simulink model "Boeing787_OldMission_ElectricalThermalHydraulicFuelECS"  (R2013a)
settings: Solver=ode23tb  SolverMode=SingleTasking  StartTime=0.0  StopTime=346  RelTol=1e-3
InitFcn:
  | load('SampleOutput.mat')
  | 
  | load('SampleFuelBurn.mat')
undefined symbols (not defined in the file or in its folder): ailerons, AirProp, B_737, elevator, FuelBurn, HydProp, landing_gear, rudder, thrust_rev
libraries: PowerFlowLib x118, simulink x20
(part 26 of 26)

== system Boeing787_OldMission_ElectricalThermalHydraulicFuelECS/ECS/Left Pack/Secondary HX (air-air)1/Air_properties_in_flows_hot_and_cold/air_properties_in_hot ==
  note: PLEASE NOTE that the air properties are based on the
      | inlet flow conditions rather than the average T and P.
      | Trying to base the properties on the average temperature
      | and even a constant pressure, the program did not work. One
      | suggestion is to average the inlet conditions with the outlet conditions
      | at a previous time step by using a memory block.x
  In_flow_bus_hot : Inport
  Bus Selector : BusSelector  OutputSignals=pres_Pa,temp_C
  C to K : Bias  Bias=273
  Cp(P,T) : Lookup_n-D  BreakpointsForDimension1=AirProp.P  BreakpointsForDimension2=AirProp.T  BreakpointsForDimension3=[1]  Table=AirProp.Cp_pt  RndMeth=Simplest  InputSameDT=on
  Cp_pt_hot : Display
  Gain : Gain  Gain=1000
  Pa to kPa : Gain  Gain=10^-3
  Pr(P,T) : Lookup_n-D  BreakpointsForDimension1=AirProp.P  BreakpointsForDimension2=AirProp.T  BreakpointsForDimension3=[1]  Table=AirProp.Pr_pt  RndMeth=Simplest  InputSameDT=on
  Pr_pt_hot : Display
  Rho(P,T) : Lookup_n-D  BreakpointsForDimension1=AirProp.P  BreakpointsForDimension2=AirProp.T  BreakpointsForDimension3=[1]  Table=AirProp.Rho_pt  RndMeth=Simplest  InputSameDT=on
  Rho_pt_hot : Display
  k(P,T) : Lookup_n-D  BreakpointsForDimension1=AirProp.P  BreakpointsForDimension2=AirProp.T  BreakpointsForDimension3=[1]  Table=AirProp.k_pt  RndMeth=Simplest  InputSameDT=on
  k_pt_hot : Display
  mu(P,T) : Lookup_n-D  BreakpointsForDimension1=AirProp.P  BreakpointsForDimension2=AirProp.T  BreakpointsForDimension3=[1]  Table=AirProp.mu_pt  RndMeth=Simplest  InputSameDT=on
  mu_pt_hot : Display
  rho_air_kgm-3 : Outport
  cp_air_Jkg-1K-1 : Outport  Port=2
  mu_air_Pa.s : Outport  Port=3
  K_air_Wm-1K-2 : Outport  Port=4
  Pr : Outport  Port=5
  wires:
  In_flow_bus_hot/1 -> Bus Selector/1
  C to K/1 -> Rho(P,T)/2, Pr(P,T)/2, k(P,T)/2, mu(P,T)/2, Cp(P,T)/2
  Bus Selector/1 -> Pa to kPa/1  "<pres_Pa>"
  Bus Selector/2 -> C to K/1  "<temp_C>"
  Pa to kPa/1 -> Rho(P,T)/1, Cp(P,T)/1, mu(P,T)/1, Pr(P,T)/1, k(P,T)/1  "press_kPa"
  Rho(P,T)/1 -> Rho_pt_hot/1, rho_air_kgm-3/1
  Pr(P,T)/1 -> Pr/1, Pr_pt_hot/1
  k(P,T)/1 -> K_air_Wm-1K-2/1, k_pt_hot/1
  mu(P,T)/1 -> mu_air_Pa.s/1, mu_pt_hot/1
  Cp(P,T)/1 -> Gain/1, Cp_pt_hot/1
  Gain/1 -> cp_air_Jkg-1K-1/1

== system Boeing787_OldMission_ElectricalThermalHydraulicFuelECS/ECS/Left Pack/Secondary HX (air-air)1/HX_and_Fin_paramters/Fin_parameters ==
  Constant : Constant  Value=l_fin
  Constant1 : Constant  Value=t_fin
  Constant2 : Constant  Value=s_fin
  Constant3 : Constant  Value=h_fin
  Constant4 : Constant  Value=K_n
  Constant5 : Constant  Value=eta_f
  Fin_length_m : Outport
  Fin_thickness_m : Outport  Port=2
  Fin_free_flow_width_m : Outport  Port=3
  Fin_free_flow_height_m : Outport  Port=4
  K_fin_Wm-1K-1 : Outport  Port=5
  Fin_eff : Outport  Port=6
  wires:
  Constant1/1 -> Fin_thickness_m/1
  Constant2/1 -> Fin_free_flow_width_m/1
  Constant3/1 -> Fin_free_flow_height_m/1
  Constant4/1 -> K_fin_Wm-1K-1/1
  Constant5/1 -> Fin_eff/1
  Constant/1 -> Fin_length_m/1

== system Boeing787_OldMission_ElectricalThermalHydraulicFuelECS/ECS/Left Pack/Secondary HX (air-air)1/HX_and_Fin_paramters/HX_parameters ==
  Other_HX_parameters : Inport
  Fin_parameters : Inport  Port=2
  Bus Selector : BusSelector  OutputSignals=L_hx
  Calculating the no of passages per fluid flow : Subsystem
  Calculating the total number of fins per HX per fluid flow : Subsystem
  Calculating total free flow area per flow : Subsystem
  Constant3 : Constant  Value=K_p
  Constant4 : Constant  Value=cp_hx
  Constant5 : Constant  Value=m_cm
  Display : Display
  Display1 : Display
  Display2 : Display
  tot_free_flow_area_m^2 : Outport
  tot_length_in_direc_of_flow_m : Outport  Port=2
  tot_no_of_fins_per_HX_per_flow : Outport  Port=3
  K_hx_Wm-1K-1 : Outport  Port=4
  cp_hx_Jkg-1K-1 : Outport  Port=5
  m_hx_kg : Outport  Port=6
  wires:
  Bus Selector/1 -> tot_length_in_direc_of_flow_m/1  "<L_hx>"
  Calculating the total number of fins per HX per fluid flow/1(Tot_no_of_fins_per_HX_per_flow) -> Display2/1, tot_no_of_fins_per_HX_per_flow/1  "N_f"
  Calculating total free flow area per flow/1(Total_free_flow_area) -> Display/1, tot_free_flow_area_m^2/1  "A"
  Calculating the no of passages per fluid flow/1(N_passages_per_flow) -> Display1/1, Calculating the total number of fins per HX per fluid flow/3(N_passages_per_flow), Calculating total free flow area per flow/3(N_passages_per_flow)
  Fin_parameters/1 -> Calculating the total number of fins per HX per fluid flow/2(Fin_parameters), Calculating total free flow area per flow/2(Fin_parameters), Calculating the no of passages per fluid flow/2(Fin_parameters)
  Other_HX_parameters/1 -> Bus Selector/1, Calculating the total number of fins per HX per fluid flow/1(Raw_HX_parameters), Calculating total free flow area per flow/1(Raw_HX_parameters), Calculating the no of passages per fluid flow/1(Raw_HX_parameters)
  Constant5/1 -> m_hx_kg/1
  Constant3/1 -> K_hx_Wm-1K-1/1
  Constant4/1 -> cp_hx_Jkg-1K-1/1

== system Boeing787_OldMission_ElectricalThermalHydraulicFuelECS/ECS/Left Pack/Secondary HX (air-air)1/HX_and_Fin_paramters/Other_HX_parameters2 ==
  Bus Creator : BusCreator
  Length in flow direction : Constant  Value=L_hx
  plate thickness : Constant  Value=t_p
  total height : Constant  Value=H_hx
  width : Constant  Value=W_hx
  Out1 : Outport
  wires:
  Bus Creator/1 -> Out1/1
  plate thickness/1 -> Bus Creator/4  "t_p"
  total height/1 -> Bus Creator/3  "H_hx"
  width/1 -> Bus Creator/2  "W_hx"
  Length in flow direction/1 -> Bus Creator/1  "L_hx"

== system Boeing787_OldMission_ElectricalThermalHydraulicFuelECS/ECS/Right Pack1/Primary HX (air-air)/Air_properties_in_flows_hot_and_cold/air_properties_in_cold ==
  note: PLEASE NOTE that the air properties are based on the
      | inlet flow conditions rather than the average T and P.
      | Trying to base the properties on the average temperature
      | and even a constant pressure, the program did not work. One
      | suggestion is to average the inlet conditions with the outlet conditions
      | at a previous time step by using a memory block.x
  In_flow_bus_cold : Inport
  Bus Selector1 : BusSelector  OutputSignals=press_Pa,temp_C
  C to K : Bias  Bias=273
  Cp(P,T) : Lookup_n-D  BreakpointsForDimension1=AirProp.P  BreakpointsForDimension2=AirProp.T  BreakpointsForDimension3=[1]  Table=AirProp.Cp_pt  RndMeth=Simplest  InputSameDT=on
  Cp_pt_hot : Display
  Gain1 : Gain  Gain=1000
  Pa to kPa : Gain  Gain=10^-3
  Pr(P,T) : Lookup_n-D  BreakpointsForDimension1=AirProp.P  BreakpointsForDimension2=AirProp.T  BreakpointsForDimension3=[1]  Table=AirProp.Pr_pt  RndMeth=Simplest  InputSameDT=on
  Pr_pt_hot : Display
  Rho(P,T) : Lookup_n-D  BreakpointsForDimension1=AirProp.P  BreakpointsForDimension2=AirProp.T  BreakpointsForDimension3=[1]  Table=AirProp.Rho_pt  RndMeth=Simplest  InputSameDT=on
  Rho_pt_hot : Display
  k(P,T) : Lookup_n-D  BreakpointsForDimension1=AirProp.P  BreakpointsForDimension2=AirProp.T  BreakpointsForDimension3=[1]  Table=AirProp.k_pt  RndMeth=Simplest  InputSameDT=on
  k_pt_hot : Display
  mu(P,T) : Lookup_n-D  BreakpointsForDimension1=AirProp.P  BreakpointsForDimension2=AirProp.T  BreakpointsForDimension3=[1]  Table=AirProp.mu_pt  RndMeth=Simplest  InputSameDT=on
  mu_pt_hot : Display
  rho_air_kgm-3 : Outport
  cp_air_Jkg-1K-1 : Outport  Port=2
  mu_air_Pa.s : Outport  Port=3
  K_air_Wm-1K-2 : Outport  Port=4
  Pr : Outport  Port=5
  wires:
  In_flow_bus_cold/1 -> Bus Selector1/1
  C to K/1 -> Rho(P,T)/2, Pr(P,T)/2, k(P,T)/2, mu(P,T)/2, Cp(P,T)/2
  Bus Selector1/1 -> Pa to kPa/1  "<press_Pa>"
  Bus Selector1/2 -> C to K/1  "<temp_C>"
  Pa to kPa/1 -> Rho(P,T)/1, Cp(P,T)/1, mu(P,T)/1, Pr(P,T)/1, k(P,T)/1  "press_kPa"
  Rho(P,T)/1 -> Rho_pt_hot/1, rho_air_kgm-3/1
  Pr(P,T)/1 -> Pr_pt_hot/1, Pr/1
  k(P,T)/1 -> k_pt_hot/1, K_air_Wm-1K-2/1
  mu(P,T)/1 -> mu_pt_hot/1, mu_air_Pa.s/1
  Cp(P,T)/1 -> Cp_pt_hot/1, Gain1/1
  Gain1/1 -> cp_air_Jkg-1K-1/1

== system Boeing787_OldMission_ElectricalThermalHydraulicFuelECS/ECS/Right Pack1/Primary HX (air-air)/Air_properties_in_flows_hot_and_cold/air_properties_in_hot ==
  note: PLEASE NOTE that the air properties are based on the
      | inlet flow conditions rather than the average T and P.
      | Trying to base the properties on the average temperature
      | and even a constant pressure, the program did not work. One
      | suggestion is to average the inlet conditions with the outlet conditions
      | at a previous time step by using a memory block.x
  In_flow_bus_hot : Inport
  Bus Selector : BusSelector  OutputSignals=pres_Pa,temp_C
  C to K : Bias  Bias=273
  Cp(P,T) : Lookup_n-D  BreakpointsForDimension1=AirProp.P  BreakpointsForDimension2=AirProp.T  BreakpointsForDimension3=[1]  Table=AirProp.Cp_pt  RndMeth=Simplest  InputSameDT=on
  Cp_pt_hot : Display
  Gain : Gain  Gain=1000
  Pa to kPa : Gain  Gain=10^-3
  Pr(P,T) : Lookup_n-D  BreakpointsForDimension1=AirProp.P  BreakpointsForDimension2=AirProp.T  BreakpointsForDimension3=[1]  Table=AirProp.Pr_pt  RndMeth=Simplest  InputSameDT=on
  Pr_pt_hot : Display
  Rho(P,T) : Lookup_n-D  BreakpointsForDimension1=AirProp.P  BreakpointsForDimension2=AirProp.T  BreakpointsForDimension3=[1]  Table=AirProp.Rho_pt  RndMeth=Simplest  InputSameDT=on
  Rho_pt_hot : Display
  k(P,T) : Lookup_n-D  BreakpointsForDimension1=AirProp.P  BreakpointsForDimension2=AirProp.T  BreakpointsForDimension3=[1]  Table=AirProp.k_pt  RndMeth=Simplest  InputSameDT=on
  k_pt_hot : Display
  mu(P,T) : Lookup_n-D  BreakpointsForDimension1=AirProp.P  BreakpointsForDimension2=AirProp.T  BreakpointsForDimension3=[1]  Table=AirProp.mu_pt  RndMeth=Simplest  InputSameDT=on
  mu_pt_hot : Display
  rho_air_kgm-3 : Outport
  cp_air_Jkg-1K-1 : Outport  Port=2
  mu_air_Pa.s : Outport  Port=3
  K_air_Wm-1K-2 : Outport  Port=4
  Pr : Outport  Port=5
  wires:
  In_flow_bus_hot/1 -> Bus Selector/1
  C to K/1 -> Rho(P,T)/2, Pr(P,T)/2, k(P,T)/2, mu(P,T)/2, Cp(P,T)/2
  Bus Selector/1 -> Pa to kPa/1  "<pres_Pa>"
  Bus Selector/2 -> C to K/1  "<temp_C>"
  Pa to kPa/1 -> Rho(P,T)/1, Cp(P,T)/1, mu(P,T)/1, Pr(P,T)/1, k(P,T)/1  "press_kPa"
  Rho(P,T)/1 -> Rho_pt_hot/1, rho_air_kgm-3/1
  Pr(P,T)/1 -> Pr/1, Pr_pt_hot/1
  k(P,T)/1 -> K_air_Wm-1K-2/1, k_pt_hot/1
  mu(P,T)/1 -> mu_air_Pa.s/1, mu_pt_hot/1
  Cp(P,T)/1 -> Gain/1, Cp_pt_hot/1
  Gain/1 -> cp_air_Jkg-1K-1/1

== system Boeing787_OldMission_ElectricalThermalHydraulicFuelECS/ECS/Right Pack1/Primary HX (air-air)/HX_and_Fin_paramters/Fin_parameters ==
  Constant : Constant  Value=l_fin
  Constant1 : Constant  Value=t_fin
  Constant2 : Constant  Value=s_fin
  Constant3 : Constant  Value=h_fin
  Constant4 : Constant  Value=K_n
  Constant5 : Constant  Value=eta_f
  Fin_length_m : Outport
  Fin_thickness_m : Outport  Port=2
  Fin_free_flow_width_m : Outport  Port=3
  Fin_free_flow_height_m : Outport  Port=4
  K_fin_Wm-1K-1 : Outport  Port=5
  Fin_eff : Outport  Port=6
  wires:
  Constant1/1 -> Fin_thickness_m/1
  Constant2/1 -> Fin_free_flow_width_m/1
  Constant3/1 -> Fin_free_flow_height_m/1
  Constant4/1 -> K_fin_Wm-1K-1/1
  Constant5/1 -> Fin_eff/1
  Constant/1 -> Fin_length_m/1

== system Boeing787_OldMission_ElectricalThermalHydraulicFuelECS/ECS/Right Pack1/Primary HX (air-air)/HX_and_Fin_paramters/HX_parameters ==
  Other_HX_parameters : Inport
  Fin_parameters : Inport  Port=2
  Bus Selector : BusSelector  OutputSignals=L_hx
  Calculating the no of passages per fluid flow : Subsystem
  Calculating the total number of fins per HX per fluid flow : Subsystem
  Calculating total free flow area per flow : Subsystem
  Constant3 : Constant  Value=K_p
  Constant4 : Constant  Value=cp_hx
  Constant5 : Constant  Value=m_cm
  Display : Display
  Display1 : Display
  Display2 : Display
  tot_free_flow_area_m^2 : Outport
  tot_length_in_direc_of_flow_m : Outport  Port=2
  tot_no_of_fins_per_HX_per_flow : Outport  Port=3
  K_hx_Wm-1K-1 : Outport  Port=4
  cp_hx_Jkg-1K-1 : Outport  Port=5
  m_hx_kg : Outport  Port=6
  wires:
  Bus Selector/1 -> tot_length_in_direc_of_flow_m/1  "<L_hx>"
  Calculating the total number of fins per HX per fluid flow/1(Tot_no_of_fins_per_HX_per_flow) -> Display2/1, tot_no_of_fins_per_HX_per_flow/1  "N_f"
  Calculating total free flow area per flow/1(Total_free_flow_area) -> Display/1, tot_free_flow_area_m^2/1  "A"
  Calculating the no of passages per fluid flow/1(N_passages_per_flow) -> Display1/1, Calculating the total number of fins per HX per fluid flow/3(N_passages_per_flow), Calculating total free flow area per flow/3(N_passages_per_flow)
  Fin_parameters/1 -> Calculating the total number of fins per HX per fluid flow/2(Fin_parameters), Calculating total free flow area per flow/2(Fin_parameters), Calculating the no of passages per fluid flow/2(Fin_parameters)
  Other_HX_parameters/1 -> Bus Selector/1, Calculating the total number of fins per HX per fluid flow/1(Raw_HX_parameters), Calculating total free flow area per flow/1(Raw_HX_parameters), Calculating the no of passages per fluid flow/1(Raw_HX_parameters)
  Constant5/1 -> m_hx_kg/1
  Constant3/1 -> K_hx_Wm-1K-1/1
  Constant4/1 -> cp_hx_Jkg-1K-1/1

== system Boeing787_OldMission_ElectricalThermalHydraulicFuelECS/ECS/Right Pack1/Primary HX (air-air)/HX_and_Fin_paramters/Other_HX_parameters2 ==
  Bus Creator : BusCreator
  Length in flow direction : Constant  Value=L_hx
  plate thickness : Constant  Value=t_p
  total height : Constant  Value=H_hx
  width : Constant  Value=W_hx
  Out1 : Outport
  wires:
  Bus Creator/1 -> Out1/1
  plate thickness/1 -> Bus Creator/4  "t_p"
  total height/1 -> Bus Creator/3  "H_hx"
  width/1 -> Bus Creator/2  "W_hx"
  Length in flow direction/1 -> Bus Creator/1  "L_hx"

== system Boeing787_OldMission_ElectricalThermalHydraulicFuelECS/ECS/Right Pack1/Secondary HX (air-air)1/Air_properties_in_flows_hot_and_cold/air_properties_in_cold ==
  note: PLEASE NOTE that the air properties are based on the
      | inlet flow conditions rather than the average T and P.
      | Trying to base the properties on the average temperature
      | and even a constant pressure, the program did not work. One
      | suggestion is to average the inlet conditions with the outlet conditions
      | at a previous time step by using a memory block.x
  In_flow_bus_cold : Inport
  Bus Selector1 : BusSelector  OutputSignals=press_Pa,temp_C
  C to K : Bias  Bias=273
  Cp(P,T) : Lookup_n-D  BreakpointsForDimension1=AirProp.P  BreakpointsForDimension2=AirProp.T  BreakpointsForDimension3=[1]  Table=AirProp.Cp_pt  RndMeth=Simplest  InputSameDT=on
  Cp_pt_hot : Display
  Gain1 : Gain  Gain=1000
  Pa to kPa : Gain  Gain=10^-3
  Pr(P,T) : Lookup_n-D  BreakpointsForDimension1=AirProp.P  BreakpointsForDimension2=AirProp.T  BreakpointsForDimension3=[1]  Table=AirProp.Pr_pt  RndMeth=Simplest  InputSameDT=on
  Pr_pt_hot : Display
  Rho(P,T) : Lookup_n-D  BreakpointsForDimension1=AirProp.P  BreakpointsForDimension2=AirProp.T  BreakpointsForDimension3=[1]  Table=AirProp.Rho_pt  RndMeth=Simplest  InputSameDT=on
  Rho_pt_hot : Display
  k(P,T) : Lookup_n-D  BreakpointsForDimension1=AirProp.P  BreakpointsForDimension2=AirProp.T  BreakpointsForDimension3=[1]  Table=AirProp.k_pt  RndMeth=Simplest  InputSameDT=on
  k_pt_hot : Display
  mu(P,T) : Lookup_n-D  BreakpointsForDimension1=AirProp.P  BreakpointsForDimension2=AirProp.T  BreakpointsForDimension3=[1]  Table=AirProp.mu_pt  RndMeth=Simplest  InputSameDT=on
  mu_pt_hot : Display
  rho_air_kgm-3 : Outport
  cp_air_Jkg-1K-1 : Outport  Port=2
  mu_air_Pa.s : Outport  Port=3
  K_air_Wm-1K-2 : Outport  Port=4
  Pr : Outport  Port=5
  wires:
  In_flow_bus_cold/1 -> Bus Selector1/1
  C to K/1 -> Rho(P,T)/2, Pr(P,T)/2, k(P,T)/2, mu(P,T)/2, Cp(P,T)/2
  Bus Selector1/1 -> Pa to kPa/1  "<press_Pa>"
  Bus Selector1/2 -> C to K/1  "<temp_C>"
  Pa to kPa/1 -> Rho(P,T)/1, Cp(P,T)/1, mu(P,T)/1, Pr(P,T)/1, k(P,T)/1  "press_kPa"
  Rho(P,T)/1 -> Rho_pt_hot/1, rho_air_kgm-3/1
  Pr(P,T)/1 -> Pr_pt_hot/1, Pr/1
  k(P,T)/1 -> k_pt_hot/1, K_air_Wm-1K-2/1
  mu(P,T)/1 -> mu_pt_hot/1, mu_air_Pa.s/1
  Cp(P,T)/1 -> Cp_pt_hot/1, Gain1/1
  Gain1/1 -> cp_air_Jkg-1K-1/1

== system Boeing787_OldMission_ElectricalThermalHydraulicFuelECS/ECS/Right Pack1/Secondary HX (air-air)1/Air_properties_in_flows_hot_and_cold/air_properties_in_hot ==
  note: PLEASE NOTE that the air properties are based on the
      | inlet flow conditions rather than the average T and P.
      | Trying to base the properties on the average temperature
      | and even a constant pressure, the program did not work. One
      | suggestion is to average the inlet conditions with the outlet conditions
      | at a previous time step by using a memory block.x
  In_flow_bus_hot : Inport
  Bus Selector : BusSelector  OutputSignals=pres_Pa,temp_C
  C to K : Bias  Bias=273
  Cp(P,T) : Lookup_n-D  BreakpointsForDimension1=AirProp.P  BreakpointsForDimension2=AirProp.T  BreakpointsForDimension3=[1]  Table=AirProp.Cp_pt  RndMeth=Simplest  InputSameDT=on
  Cp_pt_hot : Display
  Gain : Gain  Gain=1000
  Pa to kPa : Gain  Gain=10^-3
  Pr(P,T) : Lookup_n-D  BreakpointsForDimension1=AirProp.P  BreakpointsForDimension2=AirProp.T  BreakpointsForDimension3=[1]  Table=AirProp.Pr_pt  RndMeth=Simplest  InputSameDT=on
  Pr_pt_hot : Display
  Rho(P,T) : Lookup_n-D  BreakpointsForDimension1=AirProp.P  BreakpointsForDimension2=AirProp.T  BreakpointsForDimension3=[1]  Table=AirProp.Rho_pt  RndMeth=Simplest  InputSameDT=on
  Rho_pt_hot : Display
  k(P,T) : Lookup_n-D  BreakpointsForDimension1=AirProp.P  BreakpointsForDimension2=AirProp.T  BreakpointsForDimension3=[1]  Table=AirProp.k_pt  RndMeth=Simplest  InputSameDT=on
  k_pt_hot : Display
  mu(P,T) : Lookup_n-D  BreakpointsForDimension1=AirProp.P  BreakpointsForDimension2=AirProp.T  BreakpointsForDimension3=[1]  Table=AirProp.mu_pt  RndMeth=Simplest  InputSameDT=on
  mu_pt_hot : Display
  rho_air_kgm-3 : Outport
  cp_air_Jkg-1K-1 : Outport  Port=2
  mu_air_Pa.s : Outport  Port=3
  K_air_Wm-1K-2 : Outport  Port=4
  Pr : Outport  Port=5
  wires:
  In_flow_bus_hot/1 -> Bus Selector/1
  C to K/1 -> Rho(P,T)/2, Pr(P,T)/2, k(P,T)/2, mu(P,T)/2, Cp(P,T)/2
  Bus Selector/1 -> Pa to kPa/1  "<pres_Pa>"
  Bus Selector/2 -> C to K/1  "<temp_C>"
  Pa to kPa/1 -> Rho(P,T)/1, Cp(P,T)/1, mu(P,T)/1, Pr(P,T)/1, k(P,T)/1  "press_kPa"
  Rho(P,T)/1 -> Rho_pt_hot/1, rho_air_kgm-3/1
  Pr(P,T)/1 -> Pr/1, Pr_pt_hot/1
  k(P,T)/1 -> K_air_Wm-1K-2/1, k_pt_hot/1
  mu(P,T)/1 -> mu_air_Pa.s/1, mu_pt_hot/1
  Cp(P,T)/1 -> Gain/1, Cp_pt_hot/1
  Gain/1 -> cp_air_Jkg-1K-1/1

== system Boeing787_OldMission_ElectricalThermalHydraulicFuelECS/ECS/Right Pack1/Secondary HX (air-air)1/HX_and_Fin_paramters/Fin_parameters ==
  Constant : Constant  Value=l_fin
  Constant1 : Constant  Value=t_fin
  Constant2 : Constant  Value=s_fin
  Constant3 : Constant  Value=h_fin
  Constant4 : Constant  Value=K_n
  Constant5 : Constant  Value=eta_f
  Fin_length_m : Outport
  Fin_thickness_m : Outport  Port=2
  Fin_free_flow_width_m : Outport  Port=3
  Fin_free_flow_height_m : Outport  Port=4
  K_fin_Wm-1K-1 : Outport  Port=5
  Fin_eff : Outport  Port=6
  wires:
  Constant1/1 -> Fin_thickness_m/1
  Constant2/1 -> Fin_free_flow_width_m/1
  Constant3/1 -> Fin_free_flow_height_m/1
  Constant4/1 -> K_fin_Wm-1K-1/1
  Constant5/1 -> Fin_eff/1
  Constant/1 -> Fin_length_m/1

== system Boeing787_OldMission_ElectricalThermalHydraulicFuelECS/ECS/Right Pack1/Secondary HX (air-air)1/HX_and_Fin_paramters/HX_parameters ==
  Other_HX_parameters : Inport
  Fin_parameters : Inport  Port=2
  Bus Selector : BusSelector  OutputSignals=L_hx
  Calculating the no of passages per fluid flow : Subsystem
  Calculating the total number of fins per HX per fluid flow : Subsystem
  Calculating total free flow area per flow : Subsystem
  Constant3 : Constant  Value=K_p
  Constant4 : Constant  Value=cp_hx
  Constant5 : Constant  Value=m_cm
  Display : Display
  Display1 : Display
  Display2 : Display
  tot_free_flow_area_m^2 : Outport
  tot_length_in_direc_of_flow_m : Outport  Port=2
  tot_no_of_fins_per_HX_per_flow : Outport  Port=3
  K_hx_Wm-1K-1 : Outport  Port=4
  cp_hx_Jkg-1K-1 : Outport  Port=5
  m_hx_kg : Outport  Port=6
  wires:
  Bus Selector/1 -> tot_length_in_direc_of_flow_m/1  "<L_hx>"
  Calculating the total number of fins per HX per fluid flow/1(Tot_no_of_fins_per_HX_per_flow) -> Display2/1, tot_no_of_fins_per_HX_per_flow/1  "N_f"
  Calculating total free flow area per flow/1(Total_free_flow_area) -> Display/1, tot_free_flow_area_m^2/1  "A"
  Calculating the no of passages per fluid flow/1(N_passages_per_flow) -> Display1/1, Calculating the total number of fins per HX per fluid flow/3(N_passages_per_flow), Calculating total free flow area per flow/3(N_passages_per_flow)
  Fin_parameters/1 -> Calculating the total number of fins per HX per fluid flow/2(Fin_parameters), Calculating total free flow area per flow/2(Fin_parameters), Calculating the no of passages per fluid flow/2(Fin_parameters)
  Other_HX_parameters/1 -> Bus Selector/1, Calculating the total number of fins per HX per fluid flow/1(Raw_HX_parameters), Calculating total free flow area per flow/1(Raw_HX_parameters), Calculating the no of passages per fluid flow/1(Raw_HX_parameters)
  Constant5/1 -> m_hx_kg/1
  Constant3/1 -> K_hx_Wm-1K-1/1
  Constant4/1 -> cp_hx_Jkg-1K-1/1

== system Boeing787_OldMission_ElectricalThermalHydraulicFuelECS/ECS/Right Pack1/Secondary HX (air-air)1/HX_and_Fin_paramters/Other_HX_parameters2 ==
  Bus Creator : BusCreator
  Length in flow direction : Constant  Value=L_hx
  plate thickness : Constant  Value=t_p
  total height : Constant  Value=H_hx
  width : Constant  Value=W_hx
  Out1 : Outport
  wires:
  Bus Creator/1 -> Out1/1
  plate thickness/1 -> Bus Creator/4  "t_p"
  total height/1 -> Bus Creator/3  "H_hx"
  width/1 -> Bus Creator/2  "W_hx"
  Length in flow direction/1 -> Bus Creator/1  "L_hx"

== system Boeing787_OldMission_ElectricalThermalHydraulicFuelECS/ECS/Left Pack/Primary HX (air-air)/HX_and_Fin_paramters/HX_parameters/Calculating the no of passages per fluid flow ==
  Raw_HX_parameters : Inport
  Fin_parameters : Inport  Port=2
  Add : Sum  Inputs=+---
  Add1 : Sum  Inputs=+++
  Bus Selector : BusSelector  OutputSignals=H_hx,t_p
  Bus Selector1 : BusSelector  OutputSignals=h_fin,t_fin
  Display : Display
  Divide : Product  Inputs=*/
  Gain{,1..3} (4 alike) : Gain  Gain=2
  Rounding Function : Rounding  Operator=round
  N_passages_per_flow : Outport
  wires:
  Rounding Function/1 -> Display/1, N_passages_per_flow/1
  Divide/1 -> Rounding Function/1
  Add1/1 -> Divide/2
  Add/1 -> Divide/1
  Gain3/1 -> Add1/3
  Gain2/1 -> Add1/2
  Gain1/1 -> Add1/1
  Gain/1 -> Add/4
  Bus Selector/2 -> Gain3/1, Gain/1  "<t_p>"
  Bus Selector1/2 -> Gain2/1, Add/3  "<t_fin>"
  Bus Selector1/1 -> Gain1/1, Add/2  "<h_fin>"
  Bus Selector/1 -> Add/1  "<H_hx>"
  Fin_parameters/1 -> Bus Selector1/1
  Raw_HX_parameters/1 -> Bus Selector/1

== system Boeing787_OldMission_ElectricalThermalHydraulicFuelECS/ECS/Left Pack/Primary HX (air-air)/HX_and_Fin_paramters/HX_parameters/Calculating the total number of fins per HX per fluid flow ==
  Raw_HX_parameters : Inport
  Fin_parameters : Inport  Port=2
  N_passages_per_flow : Inport  Port=3
  Bus Selector : BusSelector  OutputSignals=W_hx,L_hx
  Bus Selector1 : BusSelector  OutputSignals=s_fin,t_fin,l_fin
  Divide : Product  Inputs=***//
  Rounding Function : Rounding  Operator=round
  s+t : Sum
  Tot_no_of_fins_per_HX_per_flow : Outport
  wires:
  Rounding Function/1 -> Tot_no_of_fins_per_HX_per_flow/1
  Divide/1 -> Rounding Function/1
  Bus Selector1/3 -> Divide/5  "<l_fin>"
  s+t/1 -> Divide/4  "s+t"
  N_passages_per_flow/1 -> Divide/3
  Bus Selector/2 -> Divide/2  "<L_hx>"
  Bus Selector/1 -> Divide/1  "<W_hx>"
  Bus Selector1/2 -> s+t/2  "<t_fin>"
  Bus Selector1/1 -> s+t/1  "<s_fin>"
  Fin_parameters/1 -> Bus Selector1/1
  Raw_HX_parameters/1 -> Bus Selector/1

== system Boeing787_OldMission_ElectricalThermalHydraulicFuelECS/ECS/Left Pack/Primary HX (air-air)/HX_and_Fin_paramters/HX_parameters/Calculating total free flow area per flow ==
  Raw_HX_parameters : Inport
  Fin_parameters : Inport  Port=2
  N_passages_per_flow : Inport  Port=3
  "Calculating the per fin ratio of the free flow area to the frontal area " : Subsystem
  Calculating total passages area per flow : Subsystem
  Product : Product  RndMeth=Zero
  Total_free_flow_area : Outport
  wires:
  Product/1 -> Total_free_flow_area/1
  Calculating total passages area per flow/1(total_pasages_area_per_flow) -> Product/2
  "Calculating the per fin ratio of the free flow area to the frontal area "/1(Per fin ratio of the free flow to the frontal areas) -> Product/1
  N_passages_per_flow/1 -> Calculating total passages area per flow/3(N_passages_per_flow)
  Raw_HX_parameters/1 -> Calculating total passages area per flow/2("HX_parameters ")
  Fin_parameters/1 -> Calculating total passages area per flow/1(Fin_parameters), "Calculating the per fin ratio of the free flow area to the frontal area "/1(Fin_parameters)

== system Boeing787_OldMission_ElectricalThermalHydraulicFuelECS/ECS/Left Pack/Secondary HX (air-air)1/HX_and_Fin_paramters/HX_parameters/Calculating the no of passages per fluid flow ==
  Raw_HX_parameters : Inport
  Fin_parameters : Inport  Port=2
  Add : Sum  Inputs=+---
  Add1 : Sum  Inputs=+++
  Bus Selector : BusSelector  OutputSignals=H_hx,t_p
  Bus Selector1 : BusSelector  OutputSignals=h_fin,t_fin
  Display : Display
  Divide : Product  Inputs=*/
  Gain{,1..3} (4 alike) : Gain  Gain=2
  Rounding Function : Rounding  Operator=round
  N_passages_per_flow : Outport
  wires:
  Rounding Function/1 -> Display/1, N_passages_per_flow/1
  Divide/1 -> Rounding Function/1
  Add1/1 -> Divide/2
  Add/1 -> Divide/1
  Gain3/1 -> Add1/3
  Gain2/1 -> Add1/2
  Gain1/1 -> Add1/1
  Gain/1 -> Add/4
  Bus Selector/2 -> Gain3/1, Gain/1  "<t_p>"
  Bus Selector1/2 -> Gain2/1, Add/3  "<t_fin>"
  Bus Selector1/1 -> Gain1/1, Add/2  "<h_fin>"
  Bus Selector/1 -> Add/1  "<H_hx>"
  Fin_parameters/1 -> Bus Selector1/1
  Raw_HX_parameters/1 -> Bus Selector/1

== system Boeing787_OldMission_ElectricalThermalHydraulicFuelECS/ECS/Left Pack/Secondary HX (air-air)1/HX_and_Fin_paramters/HX_parameters/Calculating the total number of fins per HX per fluid flow ==
  Raw_HX_parameters : Inport
  Fin_parameters : Inport  Port=2
  N_passages_per_flow : Inport  Port=3
  Bus Selector : BusSelector  OutputSignals=W_hx,L_hx
  Bus Selector1 : BusSelector  OutputSignals=s_fin,t_fin,l_fin
  Divide : Product  Inputs=***//
  Rounding Function : Rounding  Operator=round
  s+t : Sum
  Tot_no_of_fins_per_HX_per_flow : Outport
  wires:
  Rounding Function/1 -> Tot_no_of_fins_per_HX_per_flow/1
  Divide/1 -> Rounding Function/1
  Bus Selector1/3 -> Divide/5  "<l_fin>"
  s+t/1 -> Divide/4  "s+t"
  N_passages_per_flow/1 -> Divide/3
  Bus Selector/2 -> Divide/2  "<L_hx>"
  Bus Selector/1 -> Divide/1  "<W_hx>"
  Bus Selector1/2 -> s+t/2  "<t_fin>"
  Bus Selector1/1 -> s+t/1  "<s_fin>"
  Fin_parameters/1 -> Bus Selector1/1
  Raw_HX_parameters/1 -> Bus Selector/1

== system Boeing787_OldMission_ElectricalThermalHydraulicFuelECS/ECS/Left Pack/Secondary HX (air-air)1/HX_and_Fin_paramters/HX_parameters/Calculating total free flow area per flow ==
  Raw_HX_parameters : Inport
  Fin_parameters : Inport  Port=2
  N_passages_per_flow : Inport  Port=3
  "Calculating the per fin ratio of the free flow area to the frontal area " : Subsystem
  Calculating total passages area per flow : Subsystem
  Product : Product  RndMeth=Zero
  Total_free_flow_area : Outport
  wires:
  Product/1 -> Total_free_flow_area/1
  Calculating total passages area per flow/1(total_pasages_area_per_flow) -> Product/2
  "Calculating the per fin ratio of the free flow area to the frontal area "/1(Per fin ratio of the free flow to the frontal areas) -> Product/1
  N_passages_per_flow/1 -> Calculating total passages area per flow/3(N_passages_per_flow)
  Raw_HX_parameters/1 -> Calculating total passages area per flow/2("HX_parameters ")
  Fin_parameters/1 -> Calculating total passages area per flow/1(Fin_parameters), "Calculating the per fin ratio of the free flow area to the frontal area "/1(Fin_parameters)

== system Boeing787_OldMission_ElectricalThermalHydraulicFuelECS/ECS/Right Pack1/Primary HX (air-air)/HX_and_Fin_paramters/HX_parameters/Calculating the no of passages per fluid flow ==
  Raw_HX_parameters : Inport
  Fin_parameters : Inport  Port=2
  Add : Sum  Inputs=+---
  Add1 : Sum  Inputs=+++
  Bus Selector : BusSelector  OutputSignals=H_hx,t_p
  Bus Selector1 : BusSelector  OutputSignals=h_fin,t_fin
  Display : Display
  Divide : Product  Inputs=*/
  Gain{,1..3} (4 alike) : Gain  Gain=2
  Rounding Function : Rounding  Operator=round
  N_passages_per_flow : Outport
  wires:
  Rounding Function/1 -> Display/1, N_passages_per_flow/1
  Divide/1 -> Rounding Function/1
  Add1/1 -> Divide/2
  Add/1 -> Divide/1
  Gain3/1 -> Add1/3
  Gain2/1 -> Add1/2
  Gain1/1 -> Add1/1
  Gain/1 -> Add/4
  Bus Selector/2 -> Gain3/1, Gain/1  "<t_p>"
  Bus Selector1/2 -> Gain2/1, Add/3  "<t_fin>"
  Bus Selector1/1 -> Gain1/1, Add/2  "<h_fin>"
  Bus Selector/1 -> Add/1  "<H_hx>"
  Fin_parameters/1 -> Bus Selector1/1
  Raw_HX_parameters/1 -> Bus Selector/1

== system Boeing787_OldMission_ElectricalThermalHydraulicFuelECS/ECS/Right Pack1/Primary HX (air-air)/HX_and_Fin_paramters/HX_parameters/Calculating the total number of fins per HX per fluid flow ==
  Raw_HX_parameters : Inport
  Fin_parameters : Inport  Port=2
  N_passages_per_flow : Inport  Port=3
  Bus Selector : BusSelector  OutputSignals=W_hx,L_hx
  Bus Selector1 : BusSelector  OutputSignals=s_fin,t_fin,l_fin
  Divide : Product  Inputs=***//
  Rounding Function : Rounding  Operator=round
  s+t : Sum
  Tot_no_of_fins_per_HX_per_flow : Outport
  wires:
  Rounding Function/1 -> Tot_no_of_fins_per_HX_per_flow/1
  Divide/1 -> Rounding Function/1
  Bus Selector1/3 -> Divide/5  "<l_fin>"
  s+t/1 -> Divide/4  "s+t"
  N_passages_per_flow/1 -> Divide/3
  Bus Selector/2 -> Divide/2  "<L_hx>"
  Bus Selector/1 -> Divide/1  "<W_hx>"
  Bus Selector1/2 -> s+t/2  "<t_fin>"
  Bus Selector1/1 -> s+t/1  "<s_fin>"
  Fin_parameters/1 -> Bus Selector1/1
  Raw_HX_parameters/1 -> Bus Selector/1

== system Boeing787_OldMission_ElectricalThermalHydraulicFuelECS/ECS/Right Pack1/Primary HX (air-air)/HX_and_Fin_paramters/HX_parameters/Calculating total free flow area per flow ==
  Raw_HX_parameters : Inport
  Fin_parameters : Inport  Port=2
  N_passages_per_flow : Inport  Port=3
  "Calculating the per fin ratio of the free flow area to the frontal area " : Subsystem
  Calculating total passages area per flow : Subsystem
  Product : Product  RndMeth=Zero
  Total_free_flow_area : Outport
  wires:
  Product/1 -> Total_free_flow_area/1
  Calculating total passages area per flow/1(total_pasages_area_per_flow) -> Product/2
  "Calculating the per fin ratio of the free flow area to the frontal area "/1(Per fin ratio of the free flow to the frontal areas) -> Product/1
  N_passages_per_flow/1 -> Calculating total passages area per flow/3(N_passages_per_flow)
  Raw_HX_parameters/1 -> Calculating total passages area per flow/2("HX_parameters ")
  Fin_parameters/1 -> Calculating total passages area per flow/1(Fin_parameters), "Calculating the per fin ratio of the free flow area to the frontal area "/1(Fin_parameters)

== system Boeing787_OldMission_ElectricalThermalHydraulicFuelECS/ECS/Right Pack1/Secondary HX (air-air)1/HX_and_Fin_paramters/HX_parameters/Calculating the no of passages per fluid flow ==
  Raw_HX_parameters : Inport
  Fin_parameters : Inport  Port=2
  Add : Sum  Inputs=+---
  Add1 : Sum  Inputs=+++
  Bus Selector : BusSelector  OutputSignals=H_hx,t_p
  Bus Selector1 : BusSelector  OutputSignals=h_fin,t_fin
  Display : Display
  Divide : Product  Inputs=*/
  Gain{,1..3} (4 alike) : Gain  Gain=2
  Rounding Function : Rounding  Operator=round
  N_passages_per_flow : Outport
  wires:
  Rounding Function/1 -> Display/1, N_passages_per_flow/1
  Divide/1 -> Rounding Function/1
  Add1/1 -> Divide/2
  Add/1 -> Divide/1
  Gain3/1 -> Add1/3
  Gain2/1 -> Add1/2
  Gain1/1 -> Add1/1
  Gain/1 -> Add/4
  Bus Selector/2 -> Gain3/1, Gain/1  "<t_p>"
  Bus Selector1/2 -> Gain2/1, Add/3  "<t_fin>"
  Bus Selector1/1 -> Gain1/1, Add/2  "<h_fin>"
  Bus Selector/1 -> Add/1  "<H_hx>"
  Fin_parameters/1 -> Bus Selector1/1
  Raw_HX_parameters/1 -> Bus Selector/1

== system Boeing787_OldMission_ElectricalThermalHydraulicFuelECS/ECS/Right Pack1/Secondary HX (air-air)1/HX_and_Fin_paramters/HX_parameters/Calculating the total number of fins per HX per fluid flow ==
  Raw_HX_parameters : Inport
  Fin_parameters : Inport  Port=2
  N_passages_per_flow : Inport  Port=3
  Bus Selector : BusSelector  OutputSignals=W_hx,L_hx
  Bus Selector1 : BusSelector  OutputSignals=s_fin,t_fin,l_fin
  Divide : Product  Inputs=***//
  Rounding Function : Rounding  Operator=round
  s+t : Sum
  Tot_no_of_fins_per_HX_per_flow : Outport
  wires:
  Rounding Function/1 -> Tot_no_of_fins_per_HX_per_flow/1
  Divide/1 -> Rounding Function/1
  Bus Selector1/3 -> Divide/5  "<l_fin>"
  s+t/1 -> Divide/4  "s+t"
  N_passages_per_flow/1 -> Divide/3
  Bus Selector/2 -> Divide/2  "<L_hx>"
  Bus Selector/1 -> Divide/1  "<W_hx>"
  Bus Selector1/2 -> s+t/2  "<t_fin>"
  Bus Selector1/1 -> s+t/1  "<s_fin>"
  Fin_parameters/1 -> Bus Selector1/1
  Raw_HX_parameters/1 -> Bus Selector/1

== system Boeing787_OldMission_ElectricalThermalHydraulicFuelECS/ECS/Right Pack1/Secondary HX (air-air)1/HX_and_Fin_paramters/HX_parameters/Calculating total free flow area per flow ==
  Raw_HX_parameters : Inport
  Fin_parameters : Inport  Port=2
  N_passages_per_flow : Inport  Port=3
  "Calculating the per fin ratio of the free flow area to the frontal area " : Subsystem
  Calculating total passages area per flow : Subsystem
  Product : Product  RndMeth=Zero
  Total_free_flow_area : Outport
  wires:
  Product/1 -> Total_free_flow_area/1
  Calculating total passages area per flow/1(total_pasages_area_per_flow) -> Product/2
  "Calculating the per fin ratio of the free flow area to the frontal area "/1(Per fin ratio of the free flow to the frontal areas) -> Product/1
  N_passages_per_flow/1 -> Calculating total passages area per flow/3(N_passages_per_flow)
  Raw_HX_parameters/1 -> Calculating total passages area per flow/2("HX_parameters ")
  Fin_parameters/1 -> Calculating total passages area per flow/1(Fin_parameters), "Calculating the per fin ratio of the free flow area to the frontal area "/1(Fin_parameters)

== system Boeing787_OldMission_ElectricalThermalHydraulicFuelECS/ECS/Left Pack/Primary HX (air-air)/HX_and_Fin_paramters/HX_parameters/Calculating total free flow area per flow/Calculating the per fin ratio of the free flow area to the frontal area  ==
  Fin_parameters : Inport
  Bus Selector1 : BusSelector  OutputSignals=s_fin,t_fin,h_fin
  Divide : Product  Inputs=**//
  h+t : Sum
  s+t : Sum
  s-t : Sum  Inputs=+-
  Per fin ratio of the free flow to the frontal areas : Outport
  wires:
  Divide/1 -> Per fin ratio of the free flow to the frontal areas/1
  h+t/1 -> Divide/4  "h+t"
  s+t/1 -> Divide/3  "s+t"
  s-t/1 -> Divide/1  "s-t"
  Bus Selector1/3 -> Divide/2, h+t/2  "<h_fin>"
  Bus Selector1/2 -> h+t/1, s+t/2, s-t/2  "<t_fin>"
  Bus Selector1/1 -> s+t/1, s-t/1  "<s_fin>"
  Fin_parameters/1 -> Bus Selector1/1

== system Boeing787_OldMission_ElectricalThermalHydraulicFuelECS/ECS/Left Pack/Primary HX (air-air)/HX_and_Fin_paramters/HX_parameters/Calculating total free flow area per flow/Calculating total passages area per flow ==
  Fin_parameters : Inport
  "HX_parameters " : Inport  Port=2
  N_passages_per_flow : Inport  Port=3
  Bus Selector : BusSelector  OutputSignals=h_fin,t_fin
  Bus Selector1 : BusSelector  OutputSignals=W_hx
  Divide : Product  Inputs=***
  h+t : Sum
  total_pasages_area_per_flow : Outport
  wires:
  Divide/1 -> total_pasages_area_per_flow/1
  Bus Selector1/1 -> Divide/2  "<W_hx>"
  h+t/1 -> Divide/1
  Bus Selector/2 -> h+t/2  "<t_fin>"
  Bus Selector/1 -> h+t/1  "<h_fin>"
  N_passages_per_flow/1 -> Divide/3
  "HX_parameters "/1 -> Bus Selector1/1
  Fin_parameters/1 -> Bus Selector/1

== system Boeing787_OldMission_ElectricalThermalHydraulicFuelECS/ECS/Left Pack/Secondary HX (air-air)1/HX_and_Fin_paramters/HX_parameters/Calculating total free flow area per flow/Calculating the per fin ratio of the free flow area to the frontal area  ==
  Fin_parameters : Inport
  Bus Selector1 : BusSelector  OutputSignals=s_fin,t_fin,h_fin
  Divide : Product  Inputs=**//
  h+t : Sum
  s+t : Sum
  s-t : Sum  Inputs=+-
  Per fin ratio of the free flow to the frontal areas : Outport
  wires:
  Divide/1 -> Per fin ratio of the free flow to the frontal areas/1
  h+t/1 -> Divide/4  "h+t"
  s+t/1 -> Divide/3  "s+t"
  s-t/1 -> Divide/1  "s-t"
  Bus Selector1/3 -> Divide/2, h+t/2  "<h_fin>"
  Bus Selector1/2 -> h+t/1, s+t/2, s-t/2  "<t_fin>"
  Bus Selector1/1 -> s+t/1, s-t/1  "<s_fin>"
  Fin_parameters/1 -> Bus Selector1/1

== system Boeing787_OldMission_ElectricalThermalHydraulicFuelECS/ECS/Left Pack/Secondary HX (air-air)1/HX_and_Fin_paramters/HX_parameters/Calculating total free flow area per flow/Calculating total passages area per flow ==
  Fin_parameters : Inport
  "HX_parameters " : Inport  Port=2
  N_passages_per_flow : Inport  Port=3
  Bus Selector : BusSelector  OutputSignals=h_fin,t_fin
  Bus Selector1 : BusSelector  OutputSignals=W_hx
  Divide : Product  Inputs=***
  h+t : Sum
  total_pasages_area_per_flow : Outport
  wires:
  Divide/1 -> total_pasages_area_per_flow/1
  Bus Selector1/1 -> Divide/2  "<W_hx>"
  h+t/1 -> Divide/1
  Bus Selector/2 -> h+t/2  "<t_fin>"
  Bus Selector/1 -> h+t/1  "<h_fin>"
  N_passages_per_flow/1 -> Divide/3
  "HX_parameters "/1 -> Bus Selector1/1
  Fin_parameters/1 -> Bus Selector/1

== system Boeing787_OldMission_ElectricalThermalHydraulicFuelECS/ECS/Right Pack1/Primary HX (air-air)/HX_and_Fin_paramters/HX_parameters/Calculating total free flow area per flow/Calculating the per fin ratio of the free flow area to the frontal area  ==
  Fin_parameters : Inport
  Bus Selector1 : BusSelector  OutputSignals=s_fin,t_fin,h_fin
  Divide : Product  Inputs=**//
  h+t : Sum
  s+t : Sum
  s-t : Sum  Inputs=+-
  Per fin ratio of the free flow to the frontal areas : Outport
  wires:
  Divide/1 -> Per fin ratio of the free flow to the frontal areas/1
  h+t/1 -> Divide/4  "h+t"
  s+t/1 -> Divide/3  "s+t"
  s-t/1 -> Divide/1  "s-t"
  Bus Selector1/3 -> Divide/2, h+t/2  "<h_fin>"
  Bus Selector1/2 -> h+t/1, s+t/2, s-t/2  "<t_fin>"
  Bus Selector1/1 -> s+t/1, s-t/1  "<s_fin>"
  Fin_parameters/1 -> Bus Selector1/1

== system Boeing787_OldMission_ElectricalThermalHydraulicFuelECS/ECS/Right Pack1/Primary HX (air-air)/HX_and_Fin_paramters/HX_parameters/Calculating total free flow area per flow/Calculating total passages area per flow ==
  Fin_parameters : Inport
  "HX_parameters " : Inport  Port=2
  N_passages_per_flow : Inport  Port=3
  Bus Selector : BusSelector  OutputSignals=h_fin,t_fin
  Bus Selector1 : BusSelector  OutputSignals=W_hx
  Divide : Product  Inputs=***
  h+t : Sum
  total_pasages_area_per_flow : Outport
  wires:
  Divide/1 -> total_pasages_area_per_flow/1
  Bus Selector1/1 -> Divide/2  "<W_hx>"
  h+t/1 -> Divide/1
  Bus Selector/2 -> h+t/2  "<t_fin>"
  Bus Selector/1 -> h+t/1  "<h_fin>"
  N_passages_per_flow/1 -> Divide/3
  "HX_parameters "/1 -> Bus Selector1/1
  Fin_parameters/1 -> Bus Selector/1

== system Boeing787_OldMission_ElectricalThermalHydraulicFuelECS/ECS/Right Pack1/Secondary HX (air-air)1/HX_and_Fin_paramters/HX_parameters/Calculating total free flow area per flow/Calculating the per fin ratio of the free flow area to the frontal area  ==
  Fin_parameters : Inport
  Bus Selector1 : BusSelector  OutputSignals=s_fin,t_fin,h_fin
  Divide : Product  Inputs=**//
  h+t : Sum
  s+t : Sum
  s-t : Sum  Inputs=+-
  Per fin ratio of the free flow to the frontal areas : Outport
  wires:
  Divide/1 -> Per fin ratio of the free flow to the frontal areas/1
  h+t/1 -> Divide/4  "h+t"
  s+t/1 -> Divide/3  "s+t"
  s-t/1 -> Divide/1  "s-t"
  Bus Selector1/3 -> Divide/2, h+t/2  "<h_fin>"
  Bus Selector1/2 -> h+t/1, s+t/2, s-t/2  "<t_fin>"
  Bus Selector1/1 -> s+t/1, s-t/1  "<s_fin>"
  Fin_parameters/1 -> Bus Selector1/1

== system Boeing787_OldMission_ElectricalThermalHydraulicFuelECS/ECS/Right Pack1/Secondary HX (air-air)1/HX_and_Fin_paramters/HX_parameters/Calculating total free flow area per flow/Calculating total passages area per flow ==
  Fin_parameters : Inport
  "HX_parameters " : Inport  Port=2
  N_passages_per_flow : Inport  Port=3
  Bus Selector : BusSelector  OutputSignals=h_fin,t_fin
  Bus Selector1 : BusSelector  OutputSignals=W_hx
  Divide : Product  Inputs=***
  h+t : Sum
  total_pasages_area_per_flow : Outport
  wires:
  Divide/1 -> total_pasages_area_per_flow/1
  Bus Selector1/1 -> Divide/2  "<W_hx>"
  h+t/1 -> Divide/1
  Bus Selector/2 -> h+t/2  "<t_fin>"
  Bus Selector/1 -> h+t/1  "<h_fin>"
  N_passages_per_flow/1 -> Divide/3
  "HX_parameters "/1 -> Bus Selector1/1
  Fin_parameters/1 -> Bus Selector/1
